simulink model "exampleFlowMixerBasic"  (Simulink 7.6)
settings: Solver=ode45  SolverMode=SingleTasking  StartTime=0  StopTime=3000  FixedStep=5  MaxStep=10
libraries: carnot x5
Description:
  | This file is part of the CARNOT Blockset.
  |   CARNOT is free software: you can redistribute it and/or modify
  |   it under the terms of the GNU Lesser General Public License as
  |   published by the Free Software Foundation, either version 3
  |   of the License, or (at your option) any later version.
  |   CARNOT is distributed in the hope that it will be useful,
  |   but WITHOUT ANY WARRANTY; without even the implied warranty of
  |   MERCHANTABILITY or FITNESS FOR A PARTICULAR PURPOSE.
  |   See the GNU Lesser General Public License for more details.
  |   You should have received a copy of the GNU Lesser General Public
  |   License along with CARNOT.
  |   If not, see <http://www.gnu.org/licenses/>.
settings Model: Creator=FarG  LastModifiedBy=drhf  ExtModeTrigMode=oneshot  ExtModeArmWhenConnect=off
settings SolverCC: MaxOrder=3  ZeroCrossControl=DisableAll
settings DataIOCC: LimitDataPoints=off  SaveOutput=off  SaveTime=off
settings OptimizationCC: BlockReduction=off  BooleanDataType=off  InitFltsAndDblsToZero=on
settings DebuggingCC: SaveWithParameterizedLinksMsg=none  SignalResolutionControl=TryResolveAllWithWarning  SolverPrmCheckMsg=none  MultiTaskDSMMsg=warning  MultiTaskCondExecSysMsg=none  StrictBusMsg=None
settings HardwareCC: TargetUnknown=on
settings RTWCC: IncludeERTFirstTime=on
settings GRTTargetCC: TargetFcnLib=ansi_tfl_tmw.mat  ModelReferenceCompliant=off  ParMdlRefBuildCompliant=off  CompOptLevelCompliant=off  MatFileLogging=off

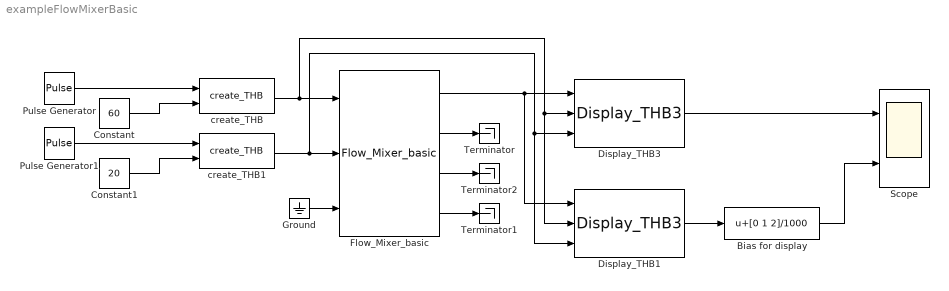
== system exampleFlowMixerBasic ==
  Bias for display : Bias  Bias=[0 1 2]/1000
  Constant : Constant  Value=60
  Constant1 : Constant  Value=20
  Display_THB1 : carnot/Outputs/Display_THB3  SystemSampleTime=-1  t=off  m=on  p=off  id=off  mix=off  d=off
  Display_THB3 : carnot/Outputs/Display_THB3  SystemSampleTime=-1  t=on  m=off  p=off  id=off  mix=off  d=off
  Flow_Mixer_basic : carnot/Basic/Hydraulics/Flow_Mixer_basic  SystemSampleTime=-1
  Ground : Ground
  Pulse Generator : DiscretePulseGenerator  PulseType=Time based  Amplitude=0.2  Period=600  PulseWidth=50
  Pulse Generator1 : DiscretePulseGenerator  PulseType=Time based  Amplitude=0.1  Period=1000  PulseWidth=50
  Scope : Scope  NumInputPorts=2
      settings: TickLabels=on  YMin=0.03~-5  YMax=0.17~5  DataFormat=Array
  Terminator : Terminator
  Terminator1 : Terminator
  Terminator2 : Terminator
  create_THB : carnot/Source/Simple/create_THB  SystemSampleTime=-1  p=1e5  fluid=Water  mix=0  dia=0.02  mID=No Pressure Drop
  create_THB1 : carnot/Source/Simple/create_THB  SystemSampleTime=-1  p=1e5  fluid=Water  mix=0  dia=0.02  mID=No Pressure Drop
  wires:
  create_THB/1 -> Flow_Mixer_basic/1, Display_THB3/2, Display_THB1/2
  create_THB1/1 -> Flow_Mixer_basic/2, Display_THB3/3, Display_THB1/3
  Ground/1 -> Flow_Mixer_basic/3
  Flow_Mixer_basic/1 -> Display_THB3/1, Display_THB1/1
  Flow_Mixer_basic/2 -> Terminator/1
  Flow_Mixer_basic/4 -> Terminator1/1
  Display_THB3/1 -> Scope/1
  Flow_Mixer_basic/3 -> Terminator2/1
  Display_THB1/1 -> Bias for display/1
  Constant/1 -> create_THB/2
  Constant1/1 -> create_THB1/2
  Pulse Generator/1 -> create_THB/1
  Pulse Generator1/1 -> create_THB1/1
  Bias for display/1 -> Scope/2
